simulink model "ddc_11bit_TestVersion_RC"  (Simulink 6.5)
settings: Solver=FixedStepDiscrete  SolverMode=SingleTasking  StartTime=0.0  StopTime=0.025  RelTol=1e-3
model workspace (MAT data in the model file):
  synDspToolFileName = 'D:\FPGA_work\kj_work\method2_Mdl\ddc_11bit_TestVersion_RC.mdl'
  synDspToolHandle : num (value not decoded)
undefined symbols (not defined in the file): syn_get_coefs
libraries: syndsplibv9 x55, syndsplibv8 x2, dspsrcs4 x1
settings Model: Creator=Administrator  LastModifiedBy=liqh  synDspstartup=OK
settings DataIOCC: SaveOutput=off  SignalLogging=off  SaveTime=off
settings OptimizationCC: InlineParams=on
settings DebuggingCC: AlgebraicLoopMsg=error  InheritedTsInSrcMsg=none

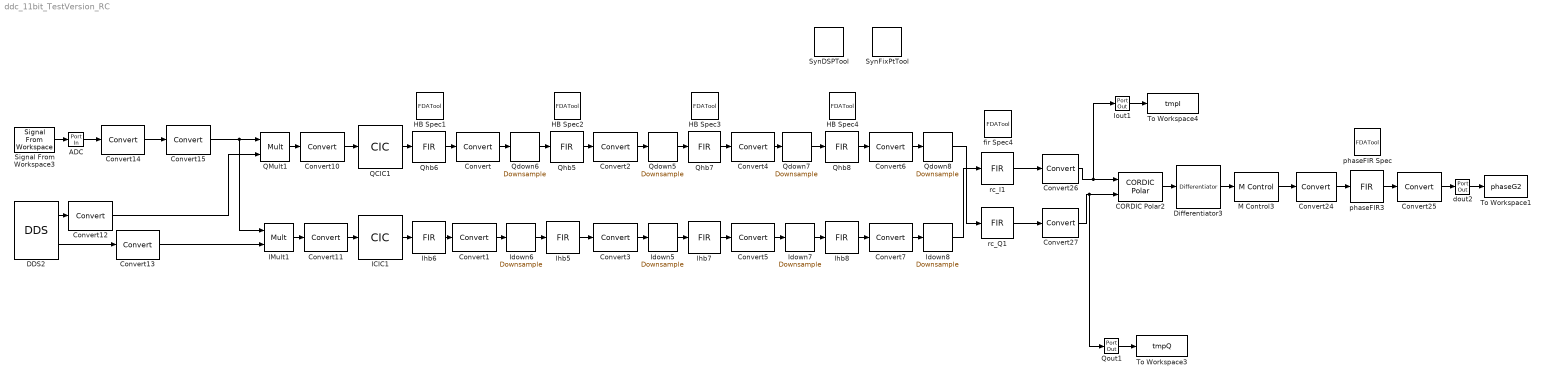
== system ddc_11bit_TestVersion_RC ==
  ADC : syndsplibv9/Ports & Subsystems/Port In  syn_out_wl=12  syn_out_fl=0  syn_out_dt=signed  syn_out_st=1/40.96e6  syn_capture=on  syn_register=on  syn_out_sat=on  syn_out_rnd=off  synBlockType=port  synLatency=1  synBlockId=0
  CORDIC Polar2 : syndsplibv9/CORDIC/CORDIC Polar  syn_polar_opr=Phase  syn_iter_nb=14  syn_out_wl=14  synBlockType=primitive  synLatency=16  synBlockId=117
  Convert : syndsplibv9/Signal Operations/Convert  syn_preshift_opr=>>  syn_preshift_bits=14  syn_preshift_val=0  syn_out_f=Specify  syn_out_wl=14  syn_out_fl=0  syn_out_dt_sync=signed  syn_out_sat=on  syn_out_rnd=Floor (Truncate)  syn_inh_port=off  syn_inh_st=off  syn_inh_stf=1  synBlockType=primitive  synLatency=0  synBlockId=4
  Convert1 : syndsplibv9/Signal Operations/Convert  syn_preshift_opr=>>  syn_preshift_bits=14  syn_preshift_val=0  syn_out_f=Specify  syn_out_wl=14  syn_out_fl=0  syn_out_dt_sync=signed  syn_out_sat=on  syn_out_rnd=Floor (Truncate)  syn_inh_port=off  syn_inh_st=off  syn_inh_stf=1  synBlockType=primitive  synLatency=0  synBlockId=4
  Convert10 : syndsplibv9/Signal Operations/Convert  syn_preshift_opr=>>  syn_preshift_bits=10  syn_preshift_val=0  syn_out_f=Specify  syn_out_wl=14  syn_out_fl=0  syn_out_dt_sync=signed  syn_out_sat=on  syn_out_rnd=Floor (Truncate)  syn_inh_port=off  syn_inh_st=off  syn_inh_stf=1  synBlockType=primitive  synLatency=0  synBlockId=4
  Convert11 : syndsplibv9/Signal Operations/Convert  syn_preshift_opr=>>  syn_preshift_bits=10  syn_preshift_val=0  syn_out_f=Specify  syn_out_wl=14  syn_out_fl=0  syn_out_dt_sync=signed  syn_out_sat=on  syn_out_rnd=Floor (Truncate)  syn_inh_port=off  syn_inh_st=off  syn_inh_stf=1  synBlockType=primitive  synLatency=0  synBlockId=4
  Convert12 : syndsplibv9/Signal Operations/Convert  syn_preshift_opr=<<  syn_preshift_bits=12  syn_preshift_val=0  syn_out_f=Specify  syn_out_wl=14  syn_out_fl=0  syn_out_dt_sync=signed  syn_out_sat=on  syn_out_rnd=Floor (Truncate)  syn_inh_port=off  syn_inh_st=off  syn_inh_stf=1  synBlockType=primitive  synLatency=0  synBlockId=4
  Convert13 : syndsplibv9/Signal Operations/Convert  syn_preshift_opr=<<  syn_preshift_bits=12  syn_preshift_val=0  syn_out_f=Specify  syn_out_wl=14  syn_out_fl=0  syn_out_dt_sync=signed  syn_out_sat=on  syn_out_rnd=Floor (Truncate)  syn_inh_port=off  syn_inh_st=off  syn_inh_stf=1  synBlockType=primitive  synLatency=0  synBlockId=4
  Convert14 : syndsplibv9/Signal Operations/Convert  syn_preshift_opr=<<  syn_preshift_bits=4  syn_preshift_val=0  syn_out_f=Specify  syn_out_wl=16  syn_out_fl=0  syn_out_dt_sync=signed  syn_out_sat=off  syn_out_rnd=Floor (Truncate)  syn_inh_port=off  syn_inh_st=off  syn_inh_stf=1  synBlockType=primitive  synLatency=0  synBlockId=4
  Convert15 : syndsplibv9/Signal Operations/Convert  syn_preshift_opr=none  syn_preshift_bits=4  syn_preshift_val=0  syn_out_f=Specify  syn_out_wl=12  syn_out_fl=0  syn_out_dt_sync=signed  syn_out_sat=on  syn_out_rnd=Floor (Truncate)  syn_inh_port=off  syn_inh_st=off  syn_inh_stf=1  synBlockType=primitive  synLatency=0  synBlockId=4
  Convert{2..7,26..27} (8 alike) : syndsplibv9/Signal Operations/Convert  syn_preshift_opr=>>  syn_preshift_bits=15  syn_preshift_val=0  syn_out_f=Specify  syn_out_wl=14  syn_out_fl=0  syn_out_dt_sync=signed  syn_out_sat=on  syn_out_rnd=Floor (Truncate)  syn_inh_port=off  syn_inh_st=off  syn_inh_stf=1  synBlockType=primitive  synLatency=0  synBlockId=4
  Convert24 : syndsplibv9/Signal Operations/Convert  syn_preshift_opr=<<  syn_preshift_bits=18  syn_preshift_val=0  syn_out_f=Specify  syn_out_wl=14  syn_out_fl=0  syn_out_dt_sync=signed  syn_out_sat=on  syn_out_rnd=Floor (Truncate)  syn_inh_port=off  syn_inh_st=off  syn_inh_stf=1  synBlockType=primitive  synLatency=0  synBlockId=4
  Convert25 : syndsplibv9/Signal Operations/Convert  syn_preshift_opr=>>  syn_preshift_bits=18  syn_preshift_val=0  syn_out_f=Specify  syn_out_wl=11  syn_out_fl=0  syn_out_dt_sync=signed  syn_out_sat=on  syn_out_rnd=Floor (Truncate)  syn_inh_port=off  syn_inh_st=off  syn_inh_stf=1  synBlockType=primitive  synLatency=0  synBlockId=4
  DDS2 : syndsplibv9/Sources/DDS  SystemSampleTime=-1  syn_dds_opr=sin&cos  syn_dds_meth=CORDIC  syn_freq_port=constant  syn_freq_val=3.89e6/40.96e6  syn_fm_port=none  syn_fm_val=4.152e6/12.288e6  syn_pm_port=none  syn_pm_val=0  syn_pdither_opr=off  syn_pdither_bits=3  syn_rst_port=off  syn_en_port=off  syn_freq_prec=2^-32  syn_phase_prec=2^-18  syn_dds_wl=18  syn_dds_st=1/40.96e6  synBlockType=custom  synLatency=20
  Differentiator3 : syndsplibv9/Filtering/Differentiator  SystemSampleTime=-1  syn_m_val=1  syn_out_f=Full Precision  syn_out_wl=16  syn_out_fl=8  syn_out_dt=signed  syn_out_sat=off  syn_out_rnd=off  syn_rst_port=off  syn_en_port=off  synBlockType=custom  synLatency=0
  HB Spec{1..4} (4 alike) : syndsplibv9/Filtering/FDATool  SystemSampleTime=-1  synBlockType=tool
  ICIC1 : syndsplibv9/Filtering/CIC  SystemSampleTime=-1  syn_cic_type=Decimator  syn_m_val=1  syn_r_val=10  syn_n_val=5  syn_out_f=Specify  syn_out_wl=14  syn_out_fl=0  syn_out_dt=signed  syn_out_sat=off  syn_out_rnd=off  syn_rst_port=off  syn_en_port=off  synBlockType=custom  synLatency=0
      settings: AttributesFormatString=0.7629394531
  IMult1 : syndsplibv9/Math Functions/Mult  syn_out_f=Full Precision  syn_out_wl=14  syn_out_fl=17  syn_out_dt=signed  syn_out_sat=on  syn_out_rnd=Round  synBlockType=primitive  synLatency=0  synBlockId=3  syn_opr_mode=1
  Idown{5..8} (4 alike) : syndsplibv9/Signal Operations/Downsample  syn_r_val=2  syn_sample_offset=0  syn_sync_mode=No Sync  synBlockType=primitive  synLatency=0  synBlockId=7
  Ihb5 : syndsplibv9/Filtering/FIR  syn_coef_vec=syn_get_coefs('HB Spec2')  syn_coef_fl=15  syn_coef_rnd=Convergent  syn_show_q=off  syn_dp_f=Algorithmic Full Precision  syn_dp_wl=16  syn_dp_fl=8  syn_dp_sat=off  syn_dp_rnd=Convergent  syn_out_f=Full Precision  syn_out_wl=14  syn_out_fl=18  syn_out_dt=signed  syn_out_sat=on  syn_out_rnd=Round  syn_rst_port=off  syn_en_port=off  synBlockType=primitive  synLatency=0  synBlockId=80
  Ihb6 : syndsplibv9/Filtering/FIR  syn_coef_vec=syn_get_coefs('HB Spec1')  syn_coef_fl=15  syn_coef_rnd=Convergent  syn_show_q=off  syn_dp_f=Algorithmic Full Precision  syn_dp_wl=16  syn_dp_fl=8  syn_dp_sat=off  syn_dp_rnd=Convergent  syn_out_f=Full Precision  syn_out_wl=16  syn_out_fl=0  syn_out_dt=signed  syn_out_sat=on  syn_out_rnd=Round  syn_rst_port=off  syn_en_port=off  synBlockType=primitive  synLatency=0  synBlockId=80
  Ihb7 : syndsplibv9/Filtering/FIR  syn_coef_vec=syn_get_coefs('HB Spec3')  syn_coef_fl=15  syn_coef_rnd=Convergent  syn_show_q=off  syn_dp_f=Algorithmic Full Precision  syn_dp_wl=16  syn_dp_fl=8  syn_dp_sat=off  syn_dp_rnd=Convergent  syn_out_f=Full Precision  syn_out_wl=14  syn_out_fl=18  syn_out_dt=signed  syn_out_sat=on  syn_out_rnd=Round  syn_rst_port=off  syn_en_port=off  synBlockType=primitive  synLatency=0  synBlockId=80
  Ihb8 : syndsplibv9/Filtering/FIR  syn_coef_vec=syn_get_coefs('HB Spec4')  syn_coef_fl=15  syn_coef_rnd=Convergent  syn_show_q=off  syn_dp_f=Algorithmic Full Precision  syn_dp_wl=16  syn_dp_fl=8  syn_dp_sat=off  syn_dp_rnd=Convergent  syn_out_f=Full Precision  syn_out_wl=14  syn_out_fl=18  syn_out_dt=signed  syn_out_sat=on  syn_out_rnd=Round  syn_rst_port=off  syn_en_port=off  synBlockType=primitive  synLatency=0  synBlockId=80
  Iout1 : syndsplibv9/Ports & Subsystems/Port Out  syn_capture=on  syn_register=on  synBlockType=port  synLatency=1  synBlockId=1
  M Control3 : syndsplibv9/Control Logic/M Control  syn_mfunc=smooth_dfai  synBlockId=1001
  QCIC1 : syndsplibv9/Filtering/CIC  SystemSampleTime=-1  syn_cic_type=Decimator  syn_m_val=1  syn_r_val=10  syn_n_val=5  syn_out_f=Specify  syn_out_wl=14  syn_out_fl=0  syn_out_dt=signed  syn_out_sat=off  syn_out_rnd=off  syn_rst_port=off  syn_en_port=off  synBlockType=custom  synLatency=0
      settings: AttributesFormatString=0.7629394531
  QMult1 : syndsplibv9/Math Functions/Mult  syn_out_f=Full Precision  syn_out_wl=14  syn_out_fl=17  syn_out_dt=signed  syn_out_sat=on  syn_out_rnd=Round  synBlockType=primitive  synLatency=0  synBlockId=3  syn_opr_mode=1
  Qdown{5..8} (4 alike) : syndsplibv9/Signal Operations/Downsample  syn_r_val=2  syn_sample_offset=0  syn_sync_mode=No Sync  synBlockType=primitive  synLatency=0  synBlockId=7
  Qhb5 : syndsplibv9/Filtering/FIR  syn_coef_vec=syn_get_coefs('HB Spec2')  syn_coef_fl=15  syn_coef_rnd=Convergent  syn_show_q=off  syn_dp_f=Algorithmic Full Precision  syn_dp_wl=16  syn_dp_fl=8  syn_dp_sat=off  syn_dp_rnd=Convergent  syn_out_f=Full Precision  syn_out_wl=14  syn_out_fl=18  syn_out_dt=signed  syn_out_sat=on  syn_out_rnd=Round  syn_rst_port=off  syn_en_port=off  synBlockType=primitive  synLatency=0  synBlockId=80
  Qhb6 : syndsplibv9/Filtering/FIR  syn_coef_vec=syn_get_coefs('HB Spec1')  syn_coef_fl=15  syn_coef_rnd=Convergent  syn_show_q=off  syn_dp_f=Algorithmic Full Precision  syn_dp_wl=16  syn_dp_fl=8  syn_dp_sat=off  syn_dp_rnd=Convergent  syn_out_f=Full Precision  syn_out_wl=16  syn_out_fl=0  syn_out_dt=signed  syn_out_sat=on  syn_out_rnd=Round  syn_rst_port=off  syn_en_port=off  synBlockType=primitive  synLatency=0  synBlockId=80
  Qhb7 : syndsplibv9/Filtering/FIR  syn_coef_vec=syn_get_coefs('HB Spec3')  syn_coef_fl=15  syn_coef_rnd=Convergent  syn_show_q=off  syn_dp_f=Algorithmic Full Precision  syn_dp_wl=16  syn_dp_fl=8  syn_dp_sat=off  syn_dp_rnd=Convergent  syn_out_f=Full Precision  syn_out_wl=14  syn_out_fl=18  syn_out_dt=signed  syn_out_sat=on  syn_out_rnd=Round  syn_rst_port=off  syn_en_port=off  synBlockType=primitive  synLatency=0  synBlockId=80
  Qhb8 : syndsplibv9/Filtering/FIR  syn_coef_vec=syn_get_coefs('HB Spec4')  syn_coef_fl=15  syn_coef_rnd=Convergent  syn_show_q=off  syn_dp_f=Algorithmic Full Precision  syn_dp_wl=16  syn_dp_fl=8  syn_dp_sat=off  syn_dp_rnd=Convergent  syn_out_f=Full Precision  syn_out_wl=14  syn_out_fl=18  syn_out_dt=signed  syn_out_sat=on  syn_out_rnd=Round  syn_rst_port=off  syn_en_port=off  synBlockType=primitive  synLatency=0  synBlockId=80
  Qout1 : syndsplibv9/Ports & Subsystems/Port Out  syn_capture=on  syn_register=on  synBlockType=port  synLatency=1  synBlockId=1
  Signal From Workspace3 : dspsrcs4/Signal From Workspace  SystemSampleTime=-1  X=sig_ddc_12bit  Ts=1/40.96e6  nsamps=1  OutputAfterFinalValue=Setting to zero  ignoreOrWarnInputAndFrameLengths=off
  SynDSPTool : syndsplibv9/SynDSPTool  SystemSampleTime=-1  synBlockType=tool  syn_dsp_mode=FPGA
  SynFixPtTool : syndsplibv9/SynFixPtTool  SystemSampleTime=-1  synBlockType=tool
  To Workspace1 : ToWorkspace  VariableName=phaseG2  SampleTime=-1  SaveFormat=Array
  To Workspace3 : ToWorkspace  VariableName=tmpQ  SampleTime=-1  SaveFormat=Array
  To Workspace4 : ToWorkspace  VariableName=tmpI  SampleTime=-1  SaveFormat=Array
  dout2 : syndsplibv9/Ports & Subsystems/Port Out  syn_capture=on  syn_register=on  synBlockType=port  synLatency=1  synBlockId=1
  fir Spec4 : syndsplibv8/Filtering/FDATool  SystemSampleTime=-1  synBlockType=tool
  phaseFIR Spec : syndsplibv8/Filtering/FDATool  SystemSampleTime=-1  synBlockType=tool
  phaseFIR3 : syndsplibv9/Filtering/FIR  syn_coef_vec=syn_get_coefs('phaseFIR Spec')  syn_coef_fl=18  syn_coef_rnd=Nearest  syn_show_q=off  syn_dp_f=Automatic  syn_dp_wl=16  syn_dp_fl=8  syn_dp_sat=off  syn_dp_rnd=Convergent  syn_out_f=Full Precision  syn_out_wl=12  syn_out_fl=16  syn_out_dt=signed  syn_out_sat=on  syn_out_rnd=Round  syn_rst_port=off  syn_en_port=off  synBlockType=primitive  synLatency=0  synBlockId=80
  rc_I1 : syndsplibv9/Filtering/FIR  syn_coef_vec=syn_get_coefs('fir Spec4')  syn_coef_fl=15  syn_coef_rnd=Convergent  syn_show_q=off  syn_dp_f=Algorithmic Full Precision  syn_dp_wl=16  syn_dp_fl=8  syn_dp_sat=off  syn_dp_rnd=Convergent  syn_out_f=Full Precision  syn_out_wl=12  syn_out_fl=16  syn_out_dt=signed  syn_out_sat=on  syn_out_rnd=Round  syn_rst_port=off  syn_en_port=off  synBlockType=primitive  synLatency=0  synBlockId=80
  rc_Q1 : syndsplibv9/Filtering/FIR  syn_coef_vec=syn_get_coefs('fir Spec4')  syn_coef_fl=15  syn_coef_rnd=Convergent  syn_show_q=off  syn_dp_f=Algorithmic Full Precision  syn_dp_wl=16  syn_dp_fl=8  syn_dp_sat=off  syn_dp_rnd=Convergent  syn_out_f=Full Precision  syn_out_wl=12  syn_out_fl=16  syn_out_dt=signed  syn_out_sat=on  syn_out_rnd=Round  syn_rst_port=off  syn_en_port=off  synBlockType=primitive  synLatency=0  synBlockId=80
  wires:
  ADC/1 -> Convert14/1
  Signal From Workspace3/1 -> ADC/1
  DDS2/1 -> Convert12/1
  DDS2/2 -> Convert13/1
  QMult1/1 -> Convert10/1
  IMult1/1 -> Convert11/1
  Qhb6/1 -> Convert/1
  Ihb6/1 -> Convert1/1
  QCIC1/1 -> Qhb6/1
  ICIC1/1 -> Ihb6/1
  Qhb5/1 -> Convert2/1
  Ihb5/1 -> Convert3/1
  Qhb7/1 -> Convert4/1
  Ihb7/1 -> Convert5/1
  Qhb8/1 -> Convert6/1
  Ihb8/1 -> Convert7/1
  Qdown6/1 -> Qhb5/1
  Idown6/1 -> Ihb5/1
  Qdown5/1 -> Qhb7/1
  Qdown7/1 -> Qhb8/1
  Idown5/1 -> Ihb7/1
  Idown7/1 -> Ihb8/1
  Convert/1 -> Qdown6/1
  Convert1/1 -> Idown6/1
  Convert2/1 -> Qdown5/1
  Convert3/1 -> Idown5/1
  Convert4/1 -> Qdown7/1
  Convert5/1 -> Idown7/1
  Convert6/1 -> Qdown8/1
  Convert7/1 -> Idown8/1
  Convert10/1 -> QCIC1/1
  Convert11/1 -> ICIC1/1
  Convert12/1 -> QMult1/2
  Convert13/1 -> IMult1/2
  Convert14/1 -> Convert15/1
  Convert15/1 -> IMult1/1, QMult1/1
  phaseFIR3/1 -> Convert25/1
  CORDIC Polar2/1 -> Differentiator3/1
  Differentiator3/1 -> M Control3/1
  M Control3/1 -> Convert24/1
  Convert24/1 -> phaseFIR3/1
  Convert25/1 -> dout2/1
  dout2/1 -> To Workspace1/1
  rc_I1/1 -> Convert26/1
  Convert26/1 -> Iout1/1, CORDIC Polar2/1
  Convert27/1 -> Qout1/1, CORDIC Polar2/2
  rc_Q1/1 -> Convert27/1
  Iout1/1 -> To Workspace4/1
  Qout1/1 -> To Workspace3/1
  Idown8/1 -> rc_I1/1
  Qdown8/1 -> rc_Q1/1
